simulink model "EX_Probe_1"  (Simulink 4.00)
settings: Solver=VariableStepDiscrete  StartTime=0.0  StopTime=10.0  FixedStep=0.01  RelTol=1e-3

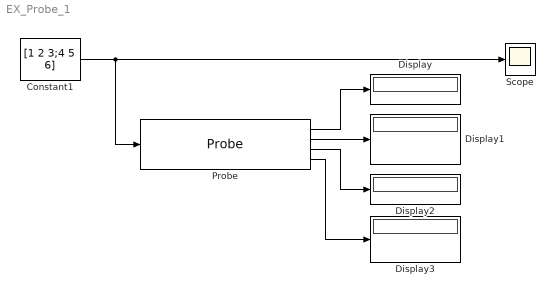
== system EX_Probe_1 ==
  Constant1 : Constant  Value=[1 2 3;4 5 6]
  Display{,1..3} (4 alike) : Display
      settings: Format=short
  Probe : Probe  ProbeWidth=on  ProbeSampleTime=on  ProbeComplexSignal=on  ProbeSignalDimensions=on
  Scope : Scope
      settings: TimeRange=10  YMin=-1  YMax=21  SaveToWorkspace=off  SaveName=ScopeData  LimitDataPoints=on  MaxDataPoints=5000
  wires:
  Constant1/1 -> Probe/1, Scope/1
  Probe/1 -> Display/1
  Probe/2 -> Display1/1
  Probe/3 -> Display2/1
  Probe/4 -> Display3/1
